simulink model "rocket_roll_plant"  (R2026a)
settings: Solver=VariableStepAuto
values from neighbouring files (symbols this model uses):
  b = 0.004    [init_roll_model.m]
  delta_max = 10*pi/180    (= 0.174532925199)    [init_roll_model.m]
  Ix = 0.003606    [init_roll_model.m]
  K_delta = 0.1    [init_roll_model.m]
  K_phi = 0.5    [init_roll_model.m]
  p_max = 0.2    [init_roll_model.m]
  phi_cmd = 0    [init_roll_model.m]
  Rate_D = 0    [init_roll_model.m]
  Rate_FF = 0    [init_roll_model.m]
  Rate_I = 0    [init_roll_model.m]
  Rate_Imax = 0.05    [init_roll_model.m]
  Rate_P = 0.5    [init_roll_model.m]
  tau_s = 0.05    [init_roll_model.m]
  Ts = 0.01    [init_roll_model.m]
  V = 20    [init_roll_model.m]
  V0 = 20    [init_roll_model.m]
undefined symbols (not defined in the file or in its folder): DiscIntNeverNeededParam
libraries: simulink x1
settings Model: Creator=vhalii  LastModifiedBy=vhalii

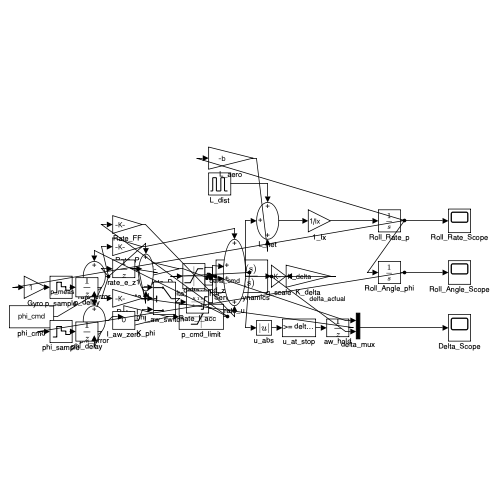
[thumbnail: Simulink's stored preview of the top-level diagram]
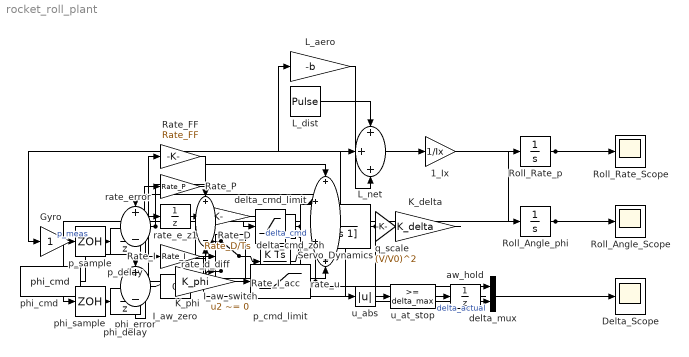
== system rocket_roll_plant ==
  1_Ix : Gain  Gain=1/Ix
  Delta_Scope : Scope
  Gyro : Gain
  I_aw_switch : Switch  Criteria=u2 ~= 0  SaturateOnIntegerOverflow=off  InputSameDT=off
  I_aw_zero : Constant  Value=0  SampleTime=Ts
  K_delta : Gain  Gain=K_delta
  K_phi : Gain  Gain=K_phi  SampleTime=Ts
  L_aero : Gain  Gain=-b
  L_dist : DiscretePulseGenerator  PulseType=Time based  Amplitude=0.01  Period=10  PulseWidth=20  PhaseDelay=1
  L_net : Sum  Inputs=+++
  Rate_D : Gain  Gain=Rate_D/Ts  SampleTime=Ts
  Rate_FF : Gain  Gain=Rate_FF  SampleTime=Ts
  Rate_I : Gain  Gain=Rate_I  SampleTime=Ts
  Rate_I_acc : DiscreteIntegrator  gainval=1  SampleTime=Ts  LimitOutput=on  UpperSaturationLimit=Rate_Imax  LowerSaturationLimit=-Rate_Imax  ICPrevOutput=DiscIntNeverNeededParam  ICPrevScaledInput=DiscIntNeverNeededParam
  Rate_P : Gain  Gain=Rate_P  SampleTime=Ts
  Roll_Angle_Scope : Scope
  Roll_Angle_phi : Integrator
  Roll_Rate_Scope : Scope
      settings: ActiveDisplayYMinimum=-0.024999999999999991  ActiveDisplayYMaximum=0.22499999999999998
  Roll_Rate_p : Integrator
  Servo_Dynamics : TransferFcn  Denominator=[tau_s 1]
  aw_hold : UnitDelay  SampleTime=Ts
  delta_cmd_limit : Saturate  UpperLimit=delta_max  LowerLimit=-delta_max  SampleTime=Ts
  delta_cmd_zoh : RateTransition  OutPortSampleTime=0
  delta_mux : Mux  Inputs=2
  p_cmd_limit : Saturate  UpperLimit=p_max  LowerLimit=-p_max  SampleTime=Ts
  p_delay : UnitDelay  SampleTime=Ts
  p_sample : ZeroOrderHold  SampleTime=Ts
  phi_cmd : Constant  Value=phi_cmd  SampleTime=Ts
  phi_delay : UnitDelay  SampleTime=Ts
  phi_error : Sum  Inputs=+-  SampleTime=Ts
  phi_sample : ZeroOrderHold  SampleTime=Ts
  q_scale : Gain  Gain=(V/V0)^2
  rate_d_diff : Sum  Inputs=+-  SampleTime=Ts
  rate_e_z1 : UnitDelay  SampleTime=Ts
  rate_error : Sum  Inputs=+-  SampleTime=Ts
  rate_u : Sum  Inputs=++++  SampleTime=Ts
  u_abs : Abs  SampleTime=Ts  SaturateOnIntegerOverflow=off
  u_at_stop : simulink/Logic and Bit Operations/Compare To Constant  relop=>=  const=delta_max  OutDataTypeStr=boolean
  wires:
  L_dist/1 -> L_net/1
  L_net/1 -> 1_Ix/1
  1_Ix/1 -> Roll_Rate_p/1
  Roll_Rate_p/1 -> Roll_Rate_Scope/1, Roll_Angle_phi/1, L_aero/1, Gyro/1
  K_delta/1 -> L_net/2
  Roll_Angle_phi/1 -> Roll_Angle_Scope/1, phi_sample/1
  phi_cmd/1 -> phi_error/1
  phi_error/1 -> K_phi/1
  K_phi/1 -> p_cmd_limit/1
  p_cmd_limit/1 -> rate_error/1, Rate_FF/1
  Servo_Dynamics/1 -> delta_mux/2, q_scale/1  "delta_actual"
  delta_mux/1 -> Delta_Scope/1
  delta_cmd_limit/1 -> delta_cmd_zoh/1  "delta_cmd"
  delta_cmd_zoh/1 -> Servo_Dynamics/1, delta_mux/1
  q_scale/1 -> K_delta/1
  L_aero/1 -> L_net/3
  p_sample/1 -> p_delay/1
  p_delay/1 -> rate_error/2
  phi_sample/1 -> phi_delay/1
  phi_delay/1 -> phi_error/2
  Gyro/1 -> p_sample/1  "p_meas"
  rate_error/1 -> Rate_P/1, rate_e_z1/1, rate_d_diff/1, Rate_I/1
  rate_e_z1/1 -> rate_d_diff/2
  rate_d_diff/1 -> Rate_D/1
  Rate_I/1 -> I_aw_switch/1
  aw_hold/1 -> I_aw_switch/2
  I_aw_zero/1 -> I_aw_switch/3
  I_aw_switch/1 -> Rate_I_acc/1
  Rate_P/1 -> rate_u/1
  Rate_I_acc/1 -> rate_u/2
  Rate_D/1 -> rate_u/3
  Rate_FF/1 -> rate_u/4
  rate_u/1 -> delta_cmd_limit/1, u_abs/1
  u_abs/1 -> u_at_stop/1
  u_at_stop/1 -> aw_hold/1
